simulink model "main"  (R2021b)
settings: Solver=VariableStepAuto  StartTime=0.0  StopTime=Inf  RelTol=1e-3
libraries: SignalEditorBlockLib x1
settings Model: Creator=Usuario  LastModifiedBy=Tiago Lucio
settings SolverCC: AlgebraicLoopSolver=TrustRegion
settings DebuggingCC: SFMachineParentedDataDiag=warning

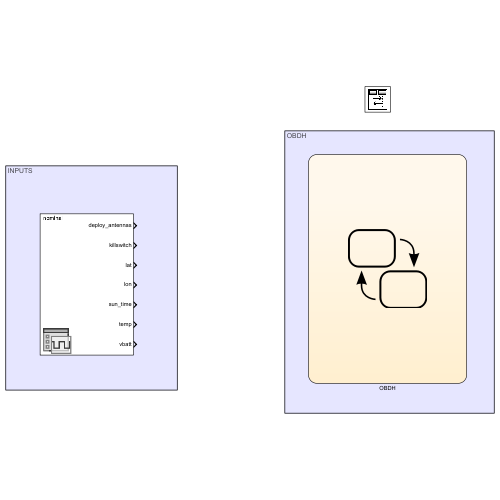
[thumbnail: Simulink's stored preview of the top-level diagram]
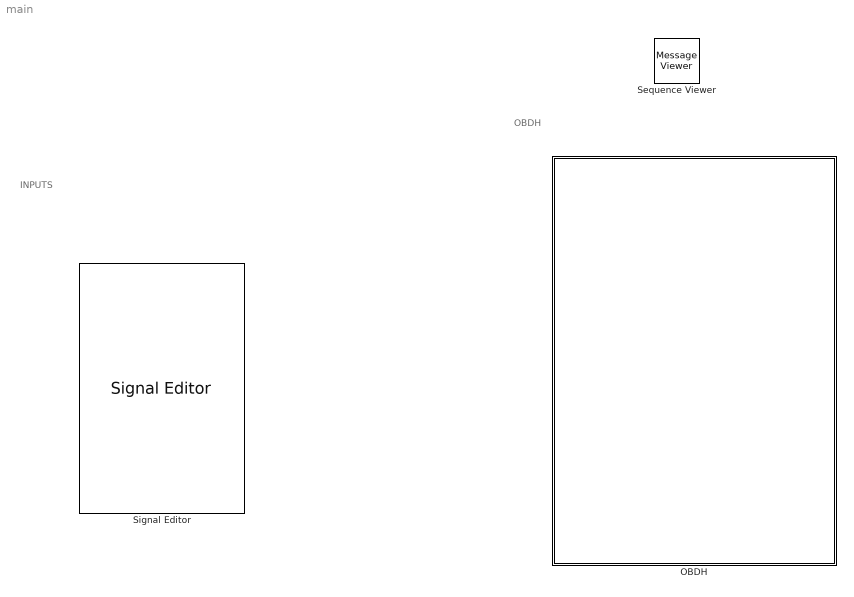
== system main ==
  note: OBDH
  note: INPUTS
  OBDH : Stateflow chart  TreatAsAtomicUnit=on
  Sequence Viewer : MessageViewer
  Signal Editor : SignalEditorBlockLib/Signal Editor  FileName=main.mat  ActiveScenario=nominal  ActiveSignal=lon  IsBus=off  OutputBusObjectStr=Bus: BusObject  SampleTime=0  Interpolate=off  ZeroCross=off  OutputAfterFinalValue=Setting to zero  Unit=degree  PreserveSignalName=on

== stateflow chart main/OBDH ==
